simulink model "clientModel"  (R2018a)
settings: Solver=VariableStepAuto  StartTime=0.0  StopTime=10  RelTol=1e-3
settings Model: Creator=hfeng  LastModifiedBy=grouleau
settings OptimizationCC: AccelVerboseBuild=on
settings RTWCC: TargetLang=C++
settings GRTTargetCC: TargetLangStandard=C++03 (ISO)  MultiInstanceERTCode=on  CodeInterfacePackaging=C++ class

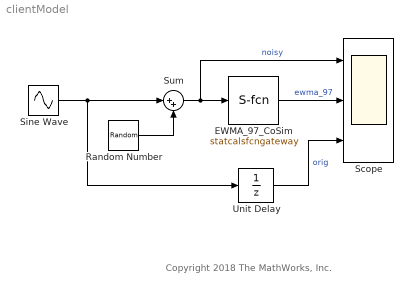
== system clientModel ==
  note: Copyright 2018 The MathWorks, Inc.
  EWMA_97_CoSim : S-Function  FunctionName=statcalsfcngateway  Parameters=hostname,portnumber,beta,initvalue,stepsize  SFunctionDeploymentMode=off  EnableBusSupport=off  mask(StatsCoSim){hostname=localhost, portnumber=8099, beta=0.97, initvalue=3, stepsize=0.01}
      mask prompts: hostname "Host name:"; portnumber "Port number:"; beta "Exponential weight:"; initvalue "Initial output value:"; stepsize "Communication step size:"
      mask help: Co-simulation gateway to stats calculation service
      mask Help: web('./statcalsfcngateway_help.html')
      mask Display: image('Simulink_Logo.png');
  Random Number : RandomNumber  Mean=[0]  Variance=[0.5]  Seed=[0]  SampleTime=0.01
  Scope : Scope  NumInputPorts=3
  Sine Wave : Sin  Amplitude=3  Phase=pi/2  SampleTime=0.01
  Sum : Sum  Inputs=|++
  Unit Delay : UnitDelay  InitialCondition=3  SampleTime=-1
  wires:
  Sine Wave/1 -> Sum/1, Unit Delay/1
  Random Number/1 -> Sum/2
  EWMA_97_CoSim/1 -> Scope/2  "ewma_97"
  Sum/1 -> EWMA_97_CoSim/1, Scope/1  "noisy"
  Unit Delay/1 -> Scope/3  "orig"
